simulink model "abssq06alg_fixpt8_32"  (R2021b)
settings: Solver=VariableStepAuto  StartTime=0.0  StopTime=99  RelTol=1e-3
undefined symbols (not defined in the file or in its folder): S, vsva2197, xcvc1902
libraries: hdlBasic x800, vmcUtilities x1
(part 1 of 6)
settings Model: Creator=abeshu  LastModifiedBy=shu_abe

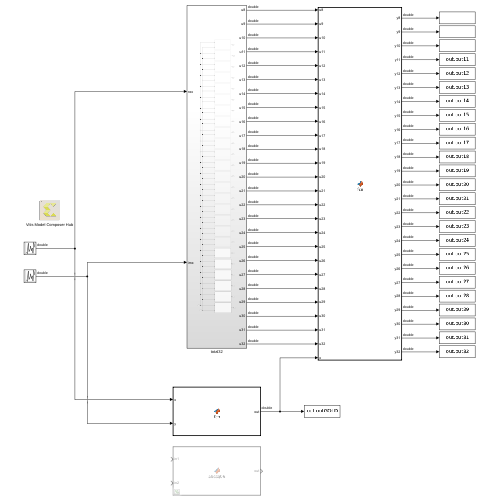
[thumbnail: Simulink's stored preview of the top-level diagram]
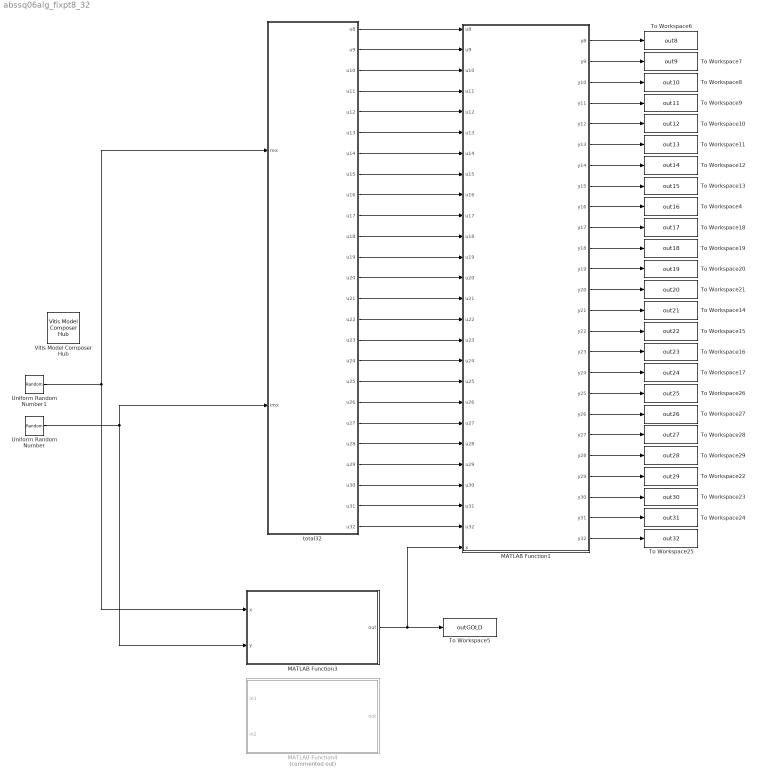
== system abssq06alg_fixpt8_32 ==
  MATLAB Function1 : MATLAB Function  TreatAsAtomicUnit=on
  MATLAB Function3 : MATLAB Function  TreatAsAtomicUnit=on
  MATLAB Function4 : MATLAB Function  Commented=on  TreatAsAtomicUnit=on
  To Workspace10 : ToWorkspace  VariableName=out12  SaveFormat=Structure With Time  SampleTime=-1
  To Workspace11 : ToWorkspace  VariableName=out13  SaveFormat=Structure With Time  SampleTime=-1
  To Workspace12 : ToWorkspace  VariableName=out14  SaveFormat=Structure With Time  SampleTime=-1
  To Workspace13 : ToWorkspace  VariableName=out15  SaveFormat=Structure With Time  SampleTime=-1
  To Workspace14 : ToWorkspace  VariableName=out21  SaveFormat=Structure With Time  SampleTime=-1
  To Workspace15 : ToWorkspace  VariableName=out22  SaveFormat=Structure With Time  SampleTime=-1
  To Workspace16 : ToWorkspace  VariableName=out23  SaveFormat=Structure With Time  SampleTime=-1
  To Workspace17 : ToWorkspace  VariableName=out24  SaveFormat=Structure With Time  SampleTime=-1
  To Workspace18 : ToWorkspace  VariableName=out17  SaveFormat=Structure With Time  SampleTime=-1
  To Workspace19 : ToWorkspace  VariableName=out18  SaveFormat=Structure With Time  SampleTime=-1
  To Workspace20 : ToWorkspace  VariableName=out19  SaveFormat=Structure With Time  SampleTime=-1
  To Workspace21 : ToWorkspace  VariableName=out20  SaveFormat=Structure With Time  SampleTime=-1
  To Workspace22 : ToWorkspace  VariableName=out29  SaveFormat=Structure With Time  SampleTime=-1
  To Workspace23 : ToWorkspace  VariableName=out30  SaveFormat=Structure With Time  SampleTime=-1
  To Workspace24 : ToWorkspace  VariableName=out31  SaveFormat=Structure With Time  SampleTime=-1
  To Workspace25 : ToWorkspace  VariableName=out32  SaveFormat=Structure With Time  SampleTime=-1
  To Workspace26 : ToWorkspace  VariableName=out25  SaveFormat=Structure With Time  SampleTime=-1
  To Workspace27 : ToWorkspace  VariableName=out26  SaveFormat=Structure With Time  SampleTime=-1
  To Workspace28 : ToWorkspace  VariableName=out27  SaveFormat=Structure With Time  SampleTime=-1
  To Workspace29 : ToWorkspace  VariableName=out28  SaveFormat=Structure With Time  SampleTime=-1
  To Workspace4 : ToWorkspace  VariableName=out16  SaveFormat=Structure With Time  SampleTime=-1
  To Workspace5 : ToWorkspace  VariableName=outGOLD  SaveFormat=Structure With Time  SampleTime=-1
  To Workspace6 : ToWorkspace  VariableName=out8  SaveFormat=Structure With Time  SampleTime=-1
  To Workspace7 : ToWorkspace  VariableName=out9  SaveFormat=Structure With Time  SampleTime=-1
  To Workspace8 : ToWorkspace  VariableName=out10  SaveFormat=Structure With Time  SampleTime=-1
  To Workspace9 : ToWorkspace  VariableName=out11  SaveFormat=Structure With Time  SampleTime=-1
  Uniform Random Number : UniformRandomNumber  Minimum=-0.9  Maximum=0.9  SampleTime=1
  Uniform Random Number1 : UniformRandomNumber  Minimum=-0.9  Maximum=0.9  Seed=1  SampleTime=1
  Vitis Model Composer Hub : vmcUtilities/Vitis Model Composer Hub  Tag=genX  CodeGeneration=off  SubsystemName=<enter or select subsystem name>  TargetDirectory=./code  ExportType=HLS C++ code  IpVendor=xilinx.com  IpLibrary=hls  IpVersion=1.0  IpHWLanguage=Verilog  AieCompilerOptions={}  CreateTestbench=off  TestbenchStackSize=10  RunAieSim=off  AieSimTimeout=50000  RunAieSimProfiling=off  LaunchVitisAnalyzer=off  PlotOutput=off  RunX86Sim=off  X86SimTimeout=10  GenHwImage=off  PlatformType=Not Specified  HwSystemType=Baremetal  HwValidationTarget=hw  ProjDevice=Alveo U250 Data Center Accelerator Card (xcu250-figd2104-2L-e)  ProjDevicePart=xcvc1902-vsva2197-2MP-e-S  SamplePeriod=-1  ClockFrequency=200  DataPathParallelism=1  xilinxfamily=virtexuplus  part=xcu250  speed=-2L-e  package=figd2104  directory=./abssq06alg_fixpt27_32  testbench=off  incr_netlist=off  synthesis_tool=Vivado  clock_wrapper=Clock Enables  dbl_ovrd=According to Block Masks  dcm_input_clock_period=10  sysclk_period=50  simulink_period=1  eval_field=0
  total32 : Subsystem
  wires:
  MATLAB Function3/1(out) -> MATLAB Function1/26(x), To Workspace5/1
  Uniform Random Number1/1 -> MATLAB Function3/1(x), total32/1(rex)
  Uniform Random Number/1 -> MATLAB Function3/2(y), total32/2(imx)
  MATLAB Function1/14(y21) -> To Workspace14/1
  MATLAB Function1/3(y10) -> To Workspace8/1
  MATLAB Function1/1(y8) -> To Workspace6/1
  MATLAB Function1/23(y30) -> To Workspace23/1
  MATLAB Function1/12(y19) -> To Workspace20/1
  MATLAB Function1/21(y28) -> To Workspace29/1
  MATLAB Function1/15(y22) -> To Workspace15/1
  MATLAB Function1/4(y11) -> To Workspace9/1
  MATLAB Function1/7(y14) -> To Workspace12/1
  MATLAB Function1/24(y31) -> To Workspace24/1
  MATLAB Function1/2(y9) -> To Workspace7/1
  MATLAB Function1/8(y15) -> To Workspace13/1
  MATLAB Function1/6(y13) -> To Workspace11/1
  MATLAB Function1/5(y12) -> To Workspace10/1
  MATLAB Function1/11(y18) -> To Workspace19/1
  MATLAB Function1/25(y32) -> To Workspace25/1
  MATLAB Function1/13(y20) -> To Workspace21/1
  MATLAB Function1/22(y29) -> To Workspace22/1
  MATLAB Function1/19(y26) -> To Workspace27/1
  MATLAB Function1/16(y23) -> To Workspace16/1
  MATLAB Function1/9(y16) -> To Workspace4/1
  MATLAB Function1/10(y17) -> To Workspace18/1
  MATLAB Function1/17(y24) -> To Workspace17/1
  MATLAB Function1/18(y25) -> To Workspace26/1
  MATLAB Function1/20(y27) -> To Workspace28/1
  total32/1(u8) -> MATLAB Function1/1(u8)
  total32/2(u9) -> MATLAB Function1/2(u9)
  total32/3(u10) -> MATLAB Function1/3(u10)
  total32/4(u11) -> MATLAB Function1/4(u11)
  total32/5(u12) -> MATLAB Function1/5(u12)
  total32/6(u13) -> MATLAB Function1/6(u13)
  total32/7(u14) -> MATLAB Function1/7(u14)
  total32/8(u15) -> MATLAB Function1/8(u15)
  total32/9(u16) -> MATLAB Function1/9(u16)
  total32/10(u17) -> MATLAB Function1/10(u17)
  total32/11(u18) -> MATLAB Function1/11(u18)
  total32/12(u19) -> MATLAB Function1/12(u19)
  total32/13(u20) -> MATLAB Function1/13(u20)
  total32/14(u21) -> MATLAB Function1/14(u21)
  total32/15(u22) -> MATLAB Function1/15(u22)
  total32/16(u23) -> MATLAB Function1/16(u23)
  total32/17(u24) -> MATLAB Function1/17(u24)
  total32/18(u25) -> MATLAB Function1/18(u25)
  total32/19(u26) -> MATLAB Function1/19(u26)
  total32/20(u27) -> MATLAB Function1/20(u27)
  total32/21(u28) -> MATLAB Function1/21(u28)
  total32/22(u29) -> MATLAB Function1/22(u29)
  total32/23(u30) -> MATLAB Function1/23(u30)
  total32/24(u31) -> MATLAB Function1/24(u31)
  total32/25(u32) -> MATLAB Function1/25(u32)

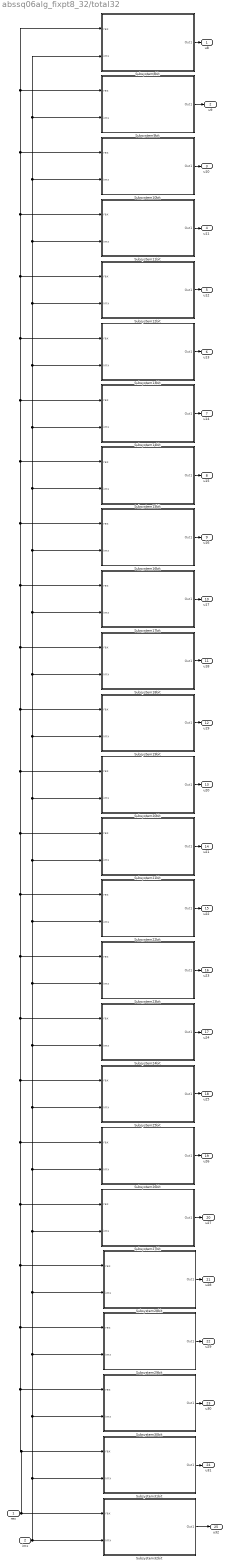
== system abssq06alg_fixpt8_32/total32 ==
  rex : Inport
  imx : Inport  Port=2
  Subsystem10bit : Subsystem
      mask Display: %%%%
  Subsystem11bit : Subsystem
      mask Display: %%%%
  Subsystem12bit : Subsystem
      mask Display: %%%%
  Subsystem13bit : Subsystem
      mask Display: %%%%
  Subsystem14bit : Subsystem
      mask Display: %%%%
  Subsystem15bit : Subsystem
      mask Display: %%%%
  Subsystem16bit : Subsystem
      mask Display: %%%%
  Subsystem17bit : Subsystem
      mask Display: %%%%
  Subsystem18bit : Subsystem
      mask Display: %%%%
  Subsystem19bit : Subsystem
      mask Display: %%%%
  Subsystem20bit : Subsystem
      mask Display: %%%%
  Subsystem21bit : Subsystem
      mask Display: %%%%
  Subsystem22bit : Subsystem
      mask Display: %%%%
  Subsystem23bit : Subsystem
      mask Display: %%%%
  Subsystem24bit : Subsystem
      mask Display: %%%%
  Subsystem25bit : Subsystem
      mask Display: %%%%
  Subsystem26bit : Subsystem
      mask Display: %%%%
  Subsystem27bit : Subsystem
      mask Display: %%%%
  Subsystem28bit : Subsystem
      mask Display: %%%%
  Subsystem29bit : Subsystem
      mask Display: %%%%
  Subsystem30bit : Subsystem
      mask Display: %%%%
  Subsystem31bit : Subsystem
      mask Display: %%%%
  Subsystem32bit : Subsystem
      mask Display: %%%%
  Subsystem8bit : Subsystem
      mask Display: %%%%
  Subsystem9bit : Subsystem
      mask Display: %%%%
  u8 : Outport
  u9 : Outport  Port=2
  u10 : Outport  Port=3
  u11 : Outport  Port=4
  u12 : Outport  Port=5
  u13 : Outport  Port=6
  u14 : Outport  Port=7
  u15 : Outport  Port=8
  u16 : Outport  Port=9
  u17 : Outport  Port=10
  u18 : Outport  Port=11
  u19 : Outport  Port=12
  u20 : Outport  Port=13
  u21 : Outport  Port=14
  u22 : Outport  Port=15
  u23 : Outport  Port=16
  u24 : Outport  Port=17
  u25 : Outport  Port=18
  u26 : Outport  Port=19
  u27 : Outport  Port=20
  u28 : Outport  Port=21
  u29 : Outport  Port=22
  u30 : Outport  Port=23
  u31 : Outport  Port=24
  u32 : Outport  Port=25
  wires:
  Subsystem17bit/1(Out1) -> u17/1
  Subsystem30bit/1(Out1) -> u30/1
  Subsystem15bit/1(Out1) -> u15/1
  Subsystem12bit/1(Out1) -> u12/1
  Subsystem14bit/1(Out1) -> u14/1
  Subsystem28bit/1(Out1) -> u28/1
  Subsystem22bit/1(Out1) -> u22/1
  Subsystem13bit/1(Out1) -> u13/1
  Subsystem21bit/1(Out1) -> u21/1
  rex/1 -> Subsystem32bit/1(rex), Subsystem31bit/1(rex), Subsystem30bit/1(rex), Subsystem29bit/1(rex), Subsystem28bit/1(rex), Subsystem27bit/1(rex), Subsystem26bit/1(rex), Subsystem25bit/1(rex), Subsystem24bit/1(rex), Subsystem23bit/1(rex), Subsystem22bit/1(rex), Subsystem21bit/1(rex), Subsystem20bit/1(rex), Subsystem19bit/1(rex), Subsystem18bit/1(rex), Subsystem17bit/1(rex), Subsystem16bit/1(rex), Subsystem15bit/1(rex), Subsystem14bit/1(rex), Subsystem13bit/1(rex), Subsystem12bit/1(rex), Subsystem11bit/1(rex), Subsystem10bit/1(rex), Subsystem9bit/1(rex), Subsystem8bit/1(rex)
  Subsystem26bit/1(Out1) -> u26/1
  Subsystem19bit/1(Out1) -> u19/1
  Subsystem10bit/1(Out1) -> u10/1
  Subsystem11bit/1(Out1) -> u11/1
  Subsystem25bit/1(Out1) -> u25/1
  Subsystem18bit/1(Out1) -> u18/1
  Subsystem20bit/1(Out1) -> u20/1
  Subsystem23bit/1(Out1) -> u23/1
  Subsystem16bit/1(Out1) -> u16/1
  Subsystem32bit/1(Out1) -> u32/1
  Subsystem27bit/1(Out1) -> u27/1
  Subsystem31bit/1(Out1) -> u31/1
  Subsystem29bit/1(Out1) -> u29/1
  Subsystem24bit/1(Out1) -> u24/1
  Subsystem8bit/1(Out1) -> u8/1
  imx/1 -> Subsystem32bit/2(imx), Subsystem31bit/2(imx), Subsystem30bit/2(imx), Subsystem29bit/2(imx), Subsystem28bit/2(imx), Subsystem27bit/2(imx), Subsystem26bit/2(imx), Subsystem25bit/2(imx), Subsystem24bit/2(imx), Subsystem23bit/2(imx), Subsystem22bit/2(imx), Subsystem21bit/2(imx), Subsystem20bit/2(imx), Subsystem19bit/2(imx), Subsystem18bit/2(imx), Subsystem17bit/2(imx), Subsystem16bit/2(imx), Subsystem15bit/2(imx), Subsystem14bit/2(imx), Subsystem13bit/2(imx), Subsystem12bit/2(imx), Subsystem11bit/2(imx), Subsystem10bit/2(imx), Subsystem9bit/2(imx), Subsystem8bit/2(imx)
  Subsystem9bit/1(Out1) -> u9/1

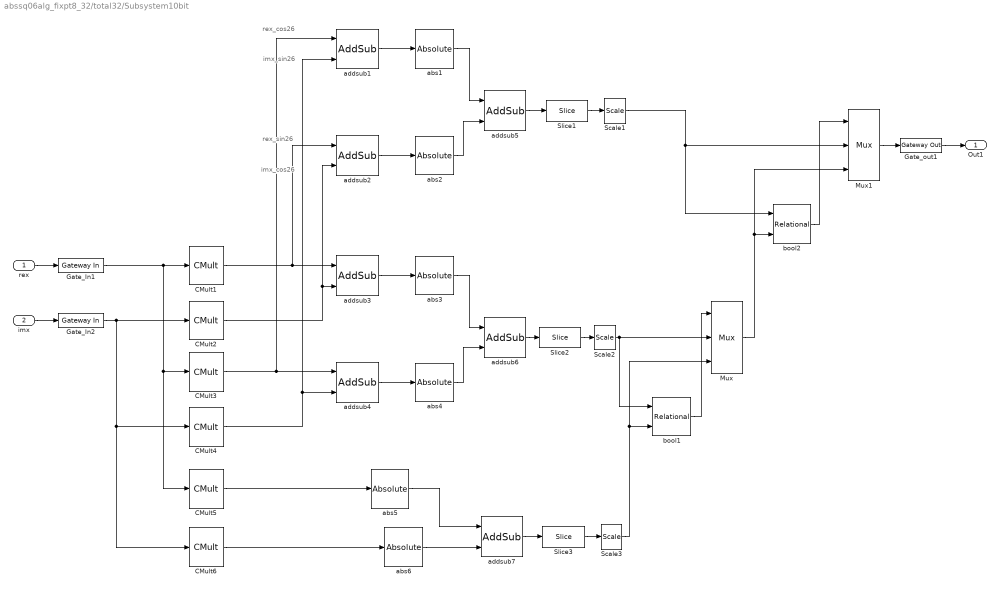
== system abssq06alg_fixpt8_32/total32/Subsystem10bit ==
  note: imx_cos26
  note: rex_sin26
  note: imx_sin26
  note: rex_cos26
  rex : Inport
  imx : Inport  Port=2
  CMult1 : hdlBasic/CMult  const=1/sqrt(2)*cos(pi/6)  gui_display_data_type=Fixed-point  const_n_bits=10  const_bin_pt=9  float_type=Double  exp_bits=8  fraction_bits=24  en=off  latency=0  precision=Full  arith_type="Signed  (2's comp)"  n_bits=16  bin_pt=14  quantization=Truncate  overflow=Wrap  use_behavioral_HDL=off  mem_type=Distributed RAM  pipeline=off  XmcBlockStatus=1  maskContainerNames=tabcontainer1  block_type=cmult  block_config=sysgen:CMult_config
      settings: infoedit=[]
  CMult2 : hdlBasic/CMult  const=1/sqrt(2)*sin(pi/6)  gui_display_data_type=Fixed-point  const_n_bits=10  const_bin_pt=9  float_type=Double  exp_bits=8  fraction_bits=24  en=off  latency=0  precision=Full  arith_type="Signed  (2's comp)"  n_bits=16  bin_pt=14  quantization=Truncate  overflow=Wrap  use_behavioral_HDL=off  mem_type=Distributed RAM  pipeline=off  XmcBlockStatus=1  maskContainerNames=tabcontainer1  block_type=cmult  block_config=sysgen:CMult_config
      settings: infoedit=[]
  CMult3 : hdlBasic/CMult  const=1/sqrt(2)*sin(pi/6)  gui_display_data_type=Fixed-point  const_n_bits=10  const_bin_pt=9  float_type=Double  exp_bits=8  fraction_bits=24  en=off  latency=0  precision=Full  arith_type="Signed  (2's comp)"  n_bits=16  bin_pt=14  quantization=Truncate  overflow=Wrap  use_behavioral_HDL=off  mem_type=Distributed RAM  pipeline=off  XmcBlockStatus=1  maskContainerNames=tabcontainer1  block_type=cmult  block_config=sysgen:CMult_config
      settings: infoedit=[]
  CMult4 : hdlBasic/CMult  const=1/sqrt(2)*cos(pi/6)  gui_display_data_type=Fixed-point  const_n_bits=10  const_bin_pt=9  float_type=Double  exp_bits=8  fraction_bits=24  en=off  latency=0  precision=Full  arith_type="Signed  (2's comp)"  n_bits=16  bin_pt=14  quantization=Truncate  overflow=Wrap  use_behavioral_HDL=off  mem_type=Distributed RAM  pipeline=off  XmcBlockStatus=1  maskContainerNames=tabcontainer1  block_type=cmult  block_config=sysgen:CMult_config
      settings: infoedit=[]
  CMult5 : hdlBasic/CMult  const=1/sqrt(2)  gui_display_data_type=Fixed-point  const_n_bits=10  const_bin_pt=9  float_type=Double  exp_bits=8  fraction_bits=24  en=off  latency=0  precision=Full  arith_type="Signed  (2's comp)"  n_bits=16  bin_pt=14  quantization=Truncate  overflow=Wrap  use_behavioral_HDL=off  mem_type=Distributed RAM  pipeline=off  XmcBlockStatus=1  maskContainerNames=tabcontainer1  block_type=cmult  block_config=sysgen:CMult_config
      settings: infoedit=[]
  CMult6 : hdlBasic/CMult  const=1/sqrt(2)  gui_display_data_type=Fixed-point  const_n_bits=10  const_bin_pt=9  float_type=Double  exp_bits=8  fraction_bits=24  en=off  latency=0  precision=Full  arith_type="Signed  (2's comp)"  n_bits=16  bin_pt=14  quantization=Truncate  overflow=Wrap  use_behavioral_HDL=off  mem_type=Distributed RAM  pipeline=off  XmcBlockStatus=1  maskContainerNames=tabcontainer1  block_type=cmult  block_config=sysgen:CMult_config
      settings: infoedit=[]
  Gate_In1 : hdlBasic/Gateway In  gui_display_data_type=Fixed-point  arith_type=Signed (2's comp)  n_bits=10  bin_pt=8  preci_type=Double  exp_width=8  frac_width=24  rows=1  columns=1  quantization="Round  (unbiased: +/- Inf)"  overflow=Saturate  period=1  UseAsADC=off  ADCChannel='1'  interface=None  automatic_assignment=on  address_offset=hex2dec('00')  intf_name=''  intf_description=''  default_value=0  timing_constraint=None  locs_specified=off  LOCs={}  io_standard={}  inherit_from_input=off  hdl_port=on  XmcBlockStatus=1  maskContainerNames=group4  block_type=gatewayin  block_config=sysgen:gateway_in_config  block_width_w=590  block_height_w=620  block_width=640  block_height=850
  Gate_In2 : hdlBasic/Gateway In  gui_display_data_type=Fixed-point  arith_type=Signed (2's comp)  n_bits=10  bin_pt=8  preci_type=Double  exp_width=8  frac_width=24  rows=1  columns=1  quantization="Round  (unbiased: +/- Inf)"  overflow=Saturate  period=1  UseAsADC=off  ADCChannel='1'  interface=None  automatic_assignment=on  address_offset=hex2dec('00')  intf_name=''  intf_description=''  default_value=0  timing_constraint=None  locs_specified=off  LOCs={}  io_standard={}  inherit_from_input=off  hdl_port=on  XmcBlockStatus=1  maskContainerNames=group4  block_type=gatewayin  block_config=sysgen:gateway_in_config  block_width_w=590  block_height_w=620  block_width=640  block_height=850
  Gate_out1 : hdlBasic/Gateway Out  inherit_from_input=off  hdl_port=on  rows=1  columns=1  UseAsDAC=off  DACChannel='1'  interface=None  automatic_assignment=on  address_offset=hex2dec('00')  intf_name=''  intf_description=''  timing_constraint=None  locs_specified=off  LOCs={}  io_standard={}  XmcBlockStatus=1  maskContainerNames=group4  block_type=gatewayout  block_config=sysgen:gateway_out_config  block_width_w=590  block_height_w=620  block_width=620  block_height=750
  Mux : hdlBasic/Mux  inputs=2  en=off  latency=0  precision=Full  arith_type=Unsigned  n_bits=16  bin_pt=14  quantization=Truncate  overflow=Wrap  XmcBlockStatus=1  maskContainerNames=tabcontainer1  block_type=mux  block_config=sysgen:Mux_config
  Mux1 : hdlBasic/Mux  inputs=2  en=off  latency=0  precision=Full  arith_type=Unsigned  n_bits=16  bin_pt=14  quantization=Truncate  overflow=Wrap  XmcBlockStatus=1  maskContainerNames=tabcontainer1  block_type=mux  block_config=sysgen:Mux_config
  Scale1 : hdlBasic/Scale  scale_factor=-9  XmcBlockStatus=1  maskContainerNames=group1  block_type=scale  block_config=sysgen:Scale_config
  Scale2 : hdlBasic/Scale  scale_factor=-9  XmcBlockStatus=1  maskContainerNames=group1  block_type=scale  block_config=sysgen:Scale_config
  Scale3 : hdlBasic/Scale  scale_factor=-9  XmcBlockStatus=1  maskContainerNames=group1  block_type=scale  block_config=sysgen:Scale_config
  Slice1 : hdlBasic/Slice  nbits=7  boolean_output=off  mode=Two Bit Locations  bit1=-5  base1=MSB of Input  bit0=8  base0=LSB of Input  XmcBlockStatus=1  maskContainerNames=group1  block_type=slice  block_config=sysgen:Slice_config
  Slice2 : hdlBasic/Slice  nbits=7  boolean_output=off  mode=Two Bit Locations  bit1=-5  base1=MSB of Input  bit0=8  base0=LSB of Input  XmcBlockStatus=1  maskContainerNames=group1  block_type=slice  block_config=sysgen:Slice_config
  Slice3 : hdlBasic/Slice  nbits=10  boolean_output=off  mode=Upper Bit Location + Width  bit1=-4  base1=MSB of Input  bit0=7  base0=LSB of Input  XmcBlockStatus=1  maskContainerNames=group1  block_type=slice  block_config=sysgen:Slice_config
  abs{1..6} (6 alike) : hdlBasic/Absolute  precision=Full  arith_type=Unsigned  n_bits=16  bin_pt=14  quantization=Truncate  overflow=Wrap  en=off  latency=0  XmcBlockStatus=1  maskContainerNames=tabcontainer1  block_type=abs  block_config=sysgen:Abs_config
  addsub1 : hdlBasic/AddSub  mode=Subtraction  use_carryin=off  use_carryout=off  en=off  latency=0  precision=Full  arith_type="Signed  (2's comp)"  n_bits=35  bin_pt=32  quantization="Round  (unbiased: +/- Inf)"  overflow=Saturate  use_behavioral_HDL=off  hw_selection=Fabric  pipelined=on  XmcBlockStatus=1  maskContainerNames=tabcontainer1  block_type=addsub  block_config=sysgen:Addsub_config
  addsub{2,4..6} (4 alike) : hdlBasic/AddSub  mode=Addition  use_carryin=off  use_carryout=off  en=off  latency=0  precision=Full  arith_type=Unsigned  n_bits=16  bin_pt=14  quantization="Round  (unbiased: +/- Inf)"  overflow=Saturate  use_behavioral_HDL=off  hw_selection=Fabric  pipelined=on  XmcBlockStatus=1  maskContainerNames=tabcontainer1  block_type=addsub  block_config=sysgen:Addsub_config
  addsub3 : hdlBasic/AddSub  mode=Subtraction  use_carryin=off  use_carryout=off  en=off  latency=0  precision=Full  arith_type="Signed  (2's comp)"  n_bits=35  bin_pt=32  quantization="Round  (unbiased: +/- Inf)"  overflow=Saturate  use_behavioral_HDL=off  hw_selection=Fabric  pipelined=on  XmcBlockStatus=1  maskContainerNames=tabcontainer1  block_type=addsub  block_config=sysgen:Addsub_config
  addsub7 : hdlBasic/AddSub  mode=Addition  use_carryin=off  use_carryout=off  en=off  latency=0  precision=Full  arith_type=Unsigned  n_bits=17  bin_pt=16  quantization="Round  (unbiased: +/- Inf)"  overflow=Saturate  use_behavioral_HDL=off  hw_selection=Fabric  pipelined=on  XmcBlockStatus=1  maskContainerNames=tabcontainer1  block_type=addsub  block_config=sysgen:Addsub_config
  bool1 : hdlBasic/Relational  mode=a<b  op_type=Bool  en=off  latency=0  XmcBlockStatus=1  maskContainerNames=tabcontainer1  block_type=relational  block_config=sysgen:Relational_config
  bool2 : hdlBasic/Relational  mode=a<b  op_type=Bool  en=off  latency=0  XmcBlockStatus=1  maskContainerNames=tabcontainer1  block_type=relational  block_config=sysgen:Relational_config
  Out1 : Outport
  wires:
  addsub3/1 -> abs3/1
  abs3/1 -> addsub6/1
  CMult1/1 -> addsub3/1, addsub2/1
  CMult2/1 -> addsub2/2, addsub3/2
  imx/1 -> Gate_In2/1
  rex/1 -> Gate_In1/1
  bool1/1 -> Mux/1
  addsub4/1 -> abs4/1
  abs4/1 -> addsub6/2
  Gate_In1/1 -> CMult1/1, CMult5/1, CMult3/1
  Gate_In2/1 -> CMult4/1, CMult6/1, CMult2/1
  CMult3/1 -> addsub4/1, addsub1/1
  CMult4/1 -> addsub4/2, addsub1/2
  addsub2/1 -> abs2/1
  abs2/1 -> addsub5/2
  addsub1/1 -> abs1/1
  abs1/1 -> addsub5/1
  Gate_out1/1 -> Out1/1
  Scale1/1 -> bool2/1, Mux1/2
  Mux/1 -> Mux1/3, bool2/2
  bool2/1 -> Mux1/1
  abs5/1 -> addsub7/1
  abs6/1 -> addsub7/2
  Mux1/1 -> Gate_out1/1
  Slice2/1 -> Scale2/1
  Slice1/1 -> Scale1/1
  Slice3/1 -> Scale3/1
  Scale2/1 -> bool1/1, Mux/2
  Scale3/1 -> Mux/3, bool1/2
  CMult5/1 -> abs5/1
  CMult6/1 -> abs6/1
  addsub5/1 -> Slice1/1
  addsub6/1 -> Slice2/1
  addsub7/1 -> Slice3/1

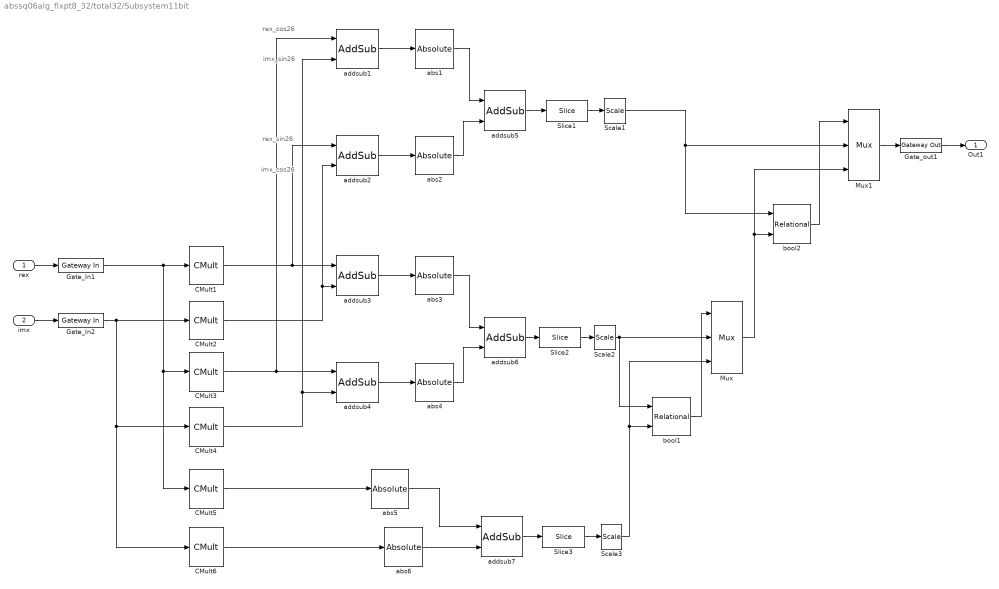
== system abssq06alg_fixpt8_32/total32/Subsystem11bit ==
  note: imx_cos26
  note: rex_sin26
  note: imx_sin26
  note: rex_cos26
  rex : Inport
  imx : Inport  Port=2
  CMult1 : hdlBasic/CMult  const=1/sqrt(2)*cos(pi/6)  gui_display_data_type=Fixed-point  const_n_bits=11  const_bin_pt=10  float_type=Double  exp_bits=8  fraction_bits=24  en=off  latency=0  precision=Full  arith_type="Signed  (2's comp)"  n_bits=16  bin_pt=14  quantization=Truncate  overflow=Wrap  use_behavioral_HDL=off  mem_type=Distributed RAM  pipeline=off  XmcBlockStatus=1  maskContainerNames=tabcontainer1  block_type=cmult  block_config=sysgen:CMult_config
      settings: infoedit=[]
  CMult2 : hdlBasic/CMult  const=1/sqrt(2)*sin(pi/6)  gui_display_data_type=Fixed-point  const_n_bits=11  const_bin_pt=10  float_type=Double  exp_bits=8  fraction_bits=24  en=off  latency=0  precision=Full  arith_type="Signed  (2's comp)"  n_bits=16  bin_pt=14  quantization=Truncate  overflow=Wrap  use_behavioral_HDL=off  mem_type=Distributed RAM  pipeline=off  XmcBlockStatus=1  maskContainerNames=tabcontainer1  block_type=cmult  block_config=sysgen:CMult_config
      settings: infoedit=[]
  CMult3 : hdlBasic/CMult  const=1/sqrt(2)*sin(pi/6)  gui_display_data_type=Fixed-point  const_n_bits=11  const_bin_pt=10  float_type=Double  exp_bits=8  fraction_bits=24  en=off  latency=0  precision=Full  arith_type="Signed  (2's comp)"  n_bits=16  bin_pt=14  quantization=Truncate  overflow=Wrap  use_behavioral_HDL=off  mem_type=Distributed RAM  pipeline=off  XmcBlockStatus=1  maskContainerNames=tabcontainer1  block_type=cmult  block_config=sysgen:CMult_config
      settings: infoedit=[]
  CMult4 : hdlBasic/CMult  const=1/sqrt(2)*cos(pi/6)  gui_display_data_type=Fixed-point  const_n_bits=11  const_bin_pt=10  float_type=Double  exp_bits=8  fraction_bits=24  en=off  latency=0  precision=Full  arith_type="Signed  (2's comp)"  n_bits=16  bin_pt=14  quantization=Truncate  overflow=Wrap  use_behavioral_HDL=off  mem_type=Distributed RAM  pipeline=off  XmcBlockStatus=1  maskContainerNames=tabcontainer1  block_type=cmult  block_config=sysgen:CMult_config
      settings: infoedit=[]
  CMult5 : hdlBasic/CMult  const=1/sqrt(2)  gui_display_data_type=Fixed-point  const_n_bits=11  const_bin_pt=10  float_type=Double  exp_bits=8  fraction_bits=24  en=off  latency=0  precision=Full  arith_type="Signed  (2's comp)"  n_bits=16  bin_pt=14  quantization=Truncate  overflow=Wrap  use_behavioral_HDL=off  mem_type=Distributed RAM  pipeline=off  XmcBlockStatus=1  maskContainerNames=tabcontainer1  block_type=cmult  block_config=sysgen:CMult_config
      settings: infoedit=[]
  CMult6 : hdlBasic/CMult  const=1/sqrt(2)  gui_display_data_type=Fixed-point  const_n_bits=11  const_bin_pt=10  float_type=Double  exp_bits=8  fraction_bits=24  en=off  latency=0  precision=Full  arith_type="Signed  (2's comp)"  n_bits=16  bin_pt=14  quantization=Truncate  overflow=Wrap  use_behavioral_HDL=off  mem_type=Distributed RAM  pipeline=off  XmcBlockStatus=1  maskContainerNames=tabcontainer1  block_type=cmult  block_config=sysgen:CMult_config
      settings: infoedit=[]
  Gate_In1 : hdlBasic/Gateway In  gui_display_data_type=Fixed-point  arith_type=Signed (2's comp)  n_bits=11  bin_pt=9  preci_type=Double  exp_width=8  frac_width=24  rows=1  columns=1  quantization="Round  (unbiased: +/- Inf)"  overflow=Saturate  period=1  UseAsADC=off  ADCChannel='1'  interface=None  automatic_assignment=on  address_offset=hex2dec('00')  intf_name=''  intf_description=''  default_value=0  timing_constraint=None  locs_specified=off  LOCs={}  io_standard={}  inherit_from_input=off  hdl_port=on  XmcBlockStatus=1  maskContainerNames=group4  block_type=gatewayin  block_config=sysgen:gateway_in_config  block_width_w=590  block_height_w=620  block_width=640  block_height=850
  Gate_In2 : hdlBasic/Gateway In  gui_display_data_type=Fixed-point  arith_type=Signed (2's comp)  n_bits=11  bin_pt=9  preci_type=Double  exp_width=8  frac_width=24  rows=1  columns=1  quantization="Round  (unbiased: +/- Inf)"  overflow=Saturate  period=1  UseAsADC=off  ADCChannel='1'  interface=None  automatic_assignment=on  address_offset=hex2dec('00')  intf_name=''  intf_description=''  default_value=0  timing_constraint=None  locs_specified=off  LOCs={}  io_standard={}  inherit_from_input=off  hdl_port=on  XmcBlockStatus=1  maskContainerNames=group4  block_type=gatewayin  block_config=sysgen:gateway_in_config  block_width_w=590  block_height_w=620  block_width=640  block_height=850
  Gate_out1 : hdlBasic/Gateway Out  inherit_from_input=off  hdl_port=on  rows=1  columns=1  UseAsDAC=off  DACChannel='1'  interface=None  automatic_assignment=on  address_offset=hex2dec('00')  intf_name=''  intf_description=''  timing_constraint=None  locs_specified=off  LOCs={}  io_standard={}  XmcBlockStatus=1  maskContainerNames=group4  block_type=gatewayout  block_config=sysgen:gateway_out_config  block_width_w=590  block_height_w=620  block_width=620  block_height=750
  Mux : hdlBasic/Mux  inputs=2  en=off  latency=0  precision=Full  arith_type=Unsigned  n_bits=16  bin_pt=14  quantization=Truncate  overflow=Wrap  XmcBlockStatus=1  maskContainerNames=tabcontainer1  block_type=mux  block_config=sysgen:Mux_config
  Mux1 : hdlBasic/Mux  inputs=2  en=off  latency=0  precision=Full  arith_type=Unsigned  n_bits=16  bin_pt=14  quantization=Truncate  overflow=Wrap  XmcBlockStatus=1  maskContainerNames=tabcontainer1  block_type=mux  block_config=sysgen:Mux_config
  Scale1 : hdlBasic/Scale  scale_factor=-10  XmcBlockStatus=1  maskContainerNames=group1  block_type=scale  block_config=sysgen:Scale_config
  Scale2 : hdlBasic/Scale  scale_factor=-10  XmcBlockStatus=1  maskContainerNames=group1  block_type=scale  block_config=sysgen:Scale_config
  Scale3 : hdlBasic/Scale  scale_factor=-10  XmcBlockStatus=1  maskContainerNames=group1  block_type=scale  block_config=sysgen:Scale_config
  Slice1 : hdlBasic/Slice  nbits=7  boolean_output=off  mode=Two Bit Locations  bit1=-5  base1=MSB of Input  bit0=9  base0=LSB of Input  XmcBlockStatus=1  maskContainerNames=group1  block_type=slice  block_config=sysgen:Slice_config
  Slice2 : hdlBasic/Slice  nbits=7  boolean_output=off  mode=Two Bit Locations  bit1=-5  base1=MSB of Input  bit0=9  base0=LSB of Input  XmcBlockStatus=1  maskContainerNames=group1  block_type=slice  block_config=sysgen:Slice_config
  Slice3 : hdlBasic/Slice  nbits=11  boolean_output=off  mode=Upper Bit Location + Width  bit1=-4  base1=MSB of Input  bit0=7  base0=LSB of Input  XmcBlockStatus=1  maskContainerNames=group1  block_type=slice  block_config=sysgen:Slice_config
  abs{1..6} (6 alike) : hdlBasic/Absolute  precision=Full  arith_type=Unsigned  n_bits=16  bin_pt=14  quantization=Truncate  overflow=Wrap  en=off  latency=0  XmcBlockStatus=1  maskContainerNames=tabcontainer1  block_type=abs  block_config=sysgen:Abs_config
  addsub1 : hdlBasic/AddSub  mode=Subtraction  use_carryin=off  use_carryout=off  en=off  latency=0  precision=Full  arith_type="Signed  (2's comp)"  n_bits=35  bin_pt=32  quantization="Round  (unbiased: +/- Inf)"  overflow=Saturate  use_behavioral_HDL=off  hw_selection=Fabric  pipelined=on  XmcBlockStatus=1  maskContainerNames=tabcontainer1  block_type=addsub  block_config=sysgen:Addsub_config
  addsub{2,4..6} (4 alike) : hdlBasic/AddSub  mode=Addition  use_carryin=off  use_carryout=off  en=off  latency=0  precision=Full  arith_type=Unsigned  n_bits=16  bin_pt=14  quantization="Round  (unbiased: +/- Inf)"  overflow=Saturate  use_behavioral_HDL=off  hw_selection=Fabric  pipelined=on  XmcBlockStatus=1  maskContainerNames=tabcontainer1  block_type=addsub  block_config=sysgen:Addsub_config
  addsub3 : hdlBasic/AddSub  mode=Subtraction  use_carryin=off  use_carryout=off  en=off  latency=0  precision=Full  arith_type="Signed  (2's comp)"  n_bits=35  bin_pt=32  quantization="Round  (unbiased: +/- Inf)"  overflow=Saturate  use_behavioral_HDL=off  hw_selection=Fabric  pipelined=on  XmcBlockStatus=1  maskContainerNames=tabcontainer1  block_type=addsub  block_config=sysgen:Addsub_config
  addsub7 : hdlBasic/AddSub  mode=Addition  use_carryin=off  use_carryout=off  en=off  latency=0  precision=Full  arith_type=Unsigned  n_bits=17  bin_pt=16  quantization="Round  (unbiased: +/- Inf)"  overflow=Saturate  use_behavioral_HDL=off  hw_selection=Fabric  pipelined=on  XmcBlockStatus=1  maskContainerNames=tabcontainer1  block_type=addsub  block_config=sysgen:Addsub_config
  bool1 : hdlBasic/Relational  mode=a<b  op_type=Bool  en=off  latency=0  XmcBlockStatus=1  maskContainerNames=tabcontainer1  block_type=relational  block_config=sysgen:Relational_config
  bool2 : hdlBasic/Relational  mode=a<b  op_type=Bool  en=off  latency=0  XmcBlockStatus=1  maskContainerNames=tabcontainer1  block_type=relational  block_config=sysgen:Relational_config
  Out1 : Outport
  wires:
  addsub3/1 -> abs3/1
  abs3/1 -> addsub6/1
  CMult1/1 -> addsub3/1, addsub2/1
  CMult2/1 -> addsub2/2, addsub3/2
  imx/1 -> Gate_In2/1
  rex/1 -> Gate_In1/1
  bool1/1 -> Mux/1
  addsub4/1 -> abs4/1
  abs4/1 -> addsub6/2
  Gate_In1/1 -> CMult1/1, CMult5/1, CMult3/1
  Gate_In2/1 -> CMult4/1, CMult6/1, CMult2/1
  CMult3/1 -> addsub4/1, addsub1/1
  CMult4/1 -> addsub4/2, addsub1/2
  addsub2/1 -> abs2/1
  abs2/1 -> addsub5/2
  addsub1/1 -> abs1/1
  abs1/1 -> addsub5/1
  Gate_out1/1 -> Out1/1
  Scale1/1 -> bool2/1, Mux1/2
  Mux/1 -> Mux1/3, bool2/2
  bool2/1 -> Mux1/1
  abs5/1 -> addsub7/1
  abs6/1 -> addsub7/2
  Mux1/1 -> Gate_out1/1
  Slice2/1 -> Scale2/1
  Slice1/1 -> Scale1/1
  Slice3/1 -> Scale3/1
  Scale2/1 -> bool1/1, Mux/2
  Scale3/1 -> Mux/3, bool1/2
  CMult5/1 -> abs5/1
  CMult6/1 -> abs6/1
  addsub5/1 -> Slice1/1
  addsub6/1 -> Slice2/1
  addsub7/1 -> Slice3/1

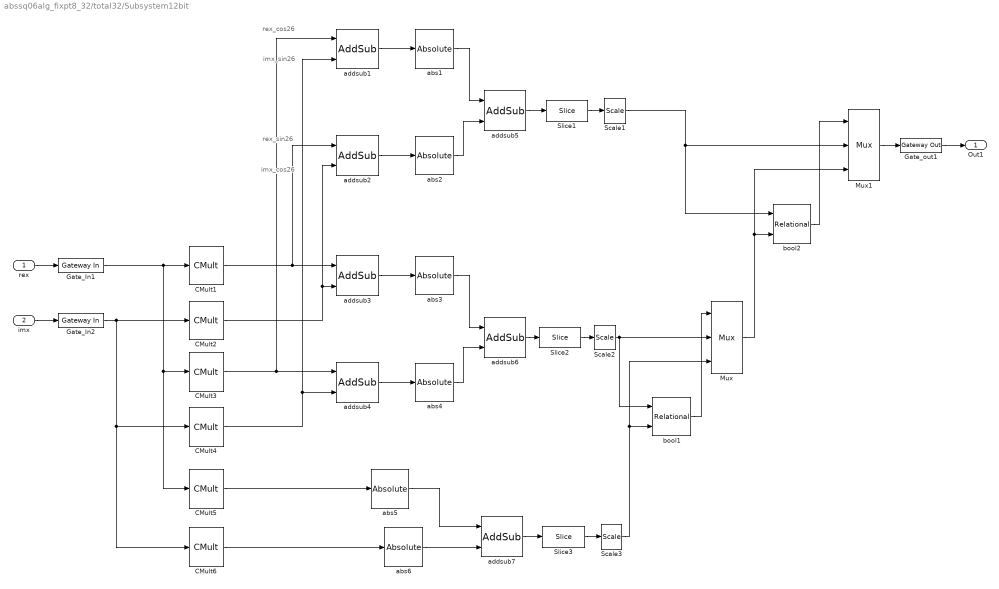
== system abssq06alg_fixpt8_32/total32/Subsystem12bit ==
  note: imx_cos26
  note: rex_sin26
  note: imx_sin26
  note: rex_cos26
  rex : Inport
  imx : Inport  Port=2
  CMult1 : hdlBasic/CMult  const=1/sqrt(2)*cos(pi/6)  gui_display_data_type=Fixed-point  const_n_bits=12  const_bin_pt=11  float_type=Double  exp_bits=8  fraction_bits=24  en=off  latency=0  precision=Full  arith_type="Signed  (2's comp)"  n_bits=16  bin_pt=14  quantization=Truncate  overflow=Wrap  use_behavioral_HDL=off  mem_type=Distributed RAM  pipeline=off  XmcBlockStatus=1  maskContainerNames=tabcontainer1  block_type=cmult  block_config=sysgen:CMult_config
      settings: infoedit=[]
  CMult2 : hdlBasic/CMult  const=1/sqrt(2)*sin(pi/6)  gui_display_data_type=Fixed-point  const_n_bits=12  const_bin_pt=11  float_type=Double  exp_bits=8  fraction_bits=24  en=off  latency=0  precision=Full  arith_type="Signed  (2's comp)"  n_bits=16  bin_pt=14  quantization=Truncate  overflow=Wrap  use_behavioral_HDL=off  mem_type=Distributed RAM  pipeline=off  XmcBlockStatus=1  maskContainerNames=tabcontainer1  block_type=cmult  block_config=sysgen:CMult_config
      settings: infoedit=[]
  CMult3 : hdlBasic/CMult  const=1/sqrt(2)*sin(pi/6)  gui_display_data_type=Fixed-point  const_n_bits=12  const_bin_pt=11  float_type=Double  exp_bits=8  fraction_bits=24  en=off  latency=0  precision=Full  arith_type="Signed  (2's comp)"  n_bits=16  bin_pt=14  quantization=Truncate  overflow=Wrap  use_behavioral_HDL=off  mem_type=Distributed RAM  pipeline=off  XmcBlockStatus=1  maskContainerNames=tabcontainer1  block_type=cmult  block_config=sysgen:CMult_config
      settings: infoedit=[]
  CMult4 : hdlBasic/CMult  const=1/sqrt(2)*cos(pi/6)  gui_display_data_type=Fixed-point  const_n_bits=12  const_bin_pt=11  float_type=Double  exp_bits=8  fraction_bits=24  en=off  latency=0  precision=Full  arith_type="Signed  (2's comp)"  n_bits=16  bin_pt=14  quantization=Truncate  overflow=Wrap  use_behavioral_HDL=off  mem_type=Distributed RAM  pipeline=off  XmcBlockStatus=1  maskContainerNames=tabcontainer1  block_type=cmult  block_config=sysgen:CMult_config
      settings: infoedit=[]
  CMult5 : hdlBasic/CMult  const=1/sqrt(2)  gui_display_data_type=Fixed-point  const_n_bits=12  const_bin_pt=11  float_type=Double  exp_bits=8  fraction_bits=24  en=off  latency=0  precision=Full  arith_type="Signed  (2's comp)"  n_bits=16  bin_pt=14  quantization=Truncate  overflow=Wrap  use_behavioral_HDL=off  mem_type=Distributed RAM  pipeline=off  XmcBlockStatus=1  maskContainerNames=tabcontainer1  block_type=cmult  block_config=sysgen:CMult_config
      settings: infoedit=[]
  CMult6 : hdlBasic/CMult  const=1/sqrt(2)  gui_display_data_type=Fixed-point  const_n_bits=12  const_bin_pt=11  float_type=Double  exp_bits=8  fraction_bits=24  en=off  latency=0  precision=Full  arith_type="Signed  (2's comp)"  n_bits=16  bin_pt=14  quantization=Truncate  overflow=Wrap  use_behavioral_HDL=off  mem_type=Distributed RAM  pipeline=off  XmcBlockStatus=1  maskContainerNames=tabcontainer1  block_type=cmult  block_config=sysgen:CMult_config
      settings: infoedit=[]
  Gate_In1 : hdlBasic/Gateway In  gui_display_data_type=Fixed-point  arith_type=Signed (2's comp)  n_bits=12  bin_pt=10  preci_type=Double  exp_width=8  frac_width=24  rows=1  columns=1  quantization="Round  (unbiased: +/- Inf)"  overflow=Saturate  period=1  UseAsADC=off  ADCChannel='1'  interface=None  automatic_assignment=on  address_offset=hex2dec('00')  intf_name=''  intf_description=''  default_value=0  timing_constraint=None  locs_specified=off  LOCs={}  io_standard={}  inherit_from_input=off  hdl_port=on  XmcBlockStatus=1  maskContainerNames=group4  block_type=gatewayin  block_config=sysgen:gateway_in_config  block_width_w=590  block_height_w=620  block_width=640  block_height=850
  Gate_In2 : hdlBasic/Gateway In  gui_display_data_type=Fixed-point  arith_type=Signed (2's comp)  n_bits=12  bin_pt=10  preci_type=Double  exp_width=8  frac_width=24  rows=1  columns=1  quantization="Round  (unbiased: +/- Inf)"  overflow=Saturate  period=1  UseAsADC=off  ADCChannel='1'  interface=None  automatic_assignment=on  address_offset=hex2dec('00')  intf_name=''  intf_description=''  default_value=0  timing_constraint=None  locs_specified=off  LOCs={}  io_standard={}  inherit_from_input=off  hdl_port=on  XmcBlockStatus=1  maskContainerNames=group4  block_type=gatewayin  block_config=sysgen:gateway_in_config  block_width_w=590  block_height_w=620  block_width=640  block_height=850
  Gate_out1 : hdlBasic/Gateway Out  inherit_from_input=off  hdl_port=on  rows=1  columns=1  UseAsDAC=off  DACChannel='1'  interface=None  automatic_assignment=on  address_offset=hex2dec('00')  intf_name=''  intf_description=''  timing_constraint=None  locs_specified=off  LOCs={}  io_standard={}  XmcBlockStatus=1  maskContainerNames=group4  block_type=gatewayout  block_config=sysgen:gateway_out_config  block_width_w=590  block_height_w=620  block_width=620  block_height=750
  Mux : hdlBasic/Mux  inputs=2  en=off  latency=0  precision=Full  arith_type=Unsigned  n_bits=16  bin_pt=14  quantization=Truncate  overflow=Wrap  XmcBlockStatus=1  maskContainerNames=tabcontainer1  block_type=mux  block_config=sysgen:Mux_config
  Mux1 : hdlBasic/Mux  inputs=2  en=off  latency=0  precision=Full  arith_type=Unsigned  n_bits=16  bin_pt=14  quantization=Truncate  overflow=Wrap  XmcBlockStatus=1  maskContainerNames=tabcontainer1  block_type=mux  block_config=sysgen:Mux_config
  Scale1 : hdlBasic/Scale  scale_factor=-11  XmcBlockStatus=1  maskContainerNames=group1  block_type=scale  block_config=sysgen:Scale_config
  Scale2 : hdlBasic/Scale  scale_factor=-11  XmcBlockStatus=1  maskContainerNames=group1  block_type=scale  block_config=sysgen:Scale_config
  Scale3 : hdlBasic/Scale  scale_factor=-11  XmcBlockStatus=1  maskContainerNames=group1  block_type=scale  block_config=sysgen:Scale_config
  Slice1 : hdlBasic/Slice  nbits=7  boolean_output=off  mode=Two Bit Locations  bit1=-5  base1=MSB of Input  bit0=10  base0=LSB of Input  XmcBlockStatus=1  maskContainerNames=group1  block_type=slice  block_config=sysgen:Slice_config
  Slice2 : hdlBasic/Slice  nbits=7  boolean_output=off  mode=Two Bit Locations  bit1=-5  base1=MSB of Input  bit0=10  base0=LSB of Input  XmcBlockStatus=1  maskContainerNames=group1  block_type=slice  block_config=sysgen:Slice_config
  Slice3 : hdlBasic/Slice  nbits=12  boolean_output=off  mode=Upper Bit Location + Width  bit1=-4  base1=MSB of Input  bit0=7  base0=LSB of Input  XmcBlockStatus=1  maskContainerNames=group1  block_type=slice  block_config=sysgen:Slice_config
  abs{1..6} (6 alike) : hdlBasic/Absolute  precision=Full  arith_type=Unsigned  n_bits=16  bin_pt=14  quantization=Truncate  overflow=Wrap  en=off  latency=0  XmcBlockStatus=1  maskContainerNames=tabcontainer1  block_type=abs  block_config=sysgen:Abs_config
  addsub1 : hdlBasic/AddSub  mode=Subtraction  use_carryin=off  use_carryout=off  en=off  latency=0  precision=Full  arith_type="Signed  (2's comp)"  n_bits=35  bin_pt=32  quantization="Round  (unbiased: +/- Inf)"  overflow=Saturate  use_behavioral_HDL=off  hw_selection=Fabric  pipelined=on  XmcBlockStatus=1  maskContainerNames=tabcontainer1  block_type=addsub  block_config=sysgen:Addsub_config
  addsub{2,4..6} (4 alike) : hdlBasic/AddSub  mode=Addition  use_carryin=off  use_carryout=off  en=off  latency=0  precision=Full  arith_type=Unsigned  n_bits=16  bin_pt=14  quantization="Round  (unbiased: +/- Inf)"  overflow=Saturate  use_behavioral_HDL=off  hw_selection=Fabric  pipelined=on  XmcBlockStatus=1  maskContainerNames=tabcontainer1  block_type=addsub  block_config=sysgen:Addsub_config
  addsub3 : hdlBasic/AddSub  mode=Subtraction  use_carryin=off  use_carryout=off  en=off  latency=0  precision=Full  arith_type="Signed  (2's comp)"  n_bits=35  bin_pt=32  quantization="Round  (unbiased: +/- Inf)"  overflow=Saturate  use_behavioral_HDL=off  hw_selection=Fabric  pipelined=on  XmcBlockStatus=1  maskContainerNames=tabcontainer1  block_type=addsub  block_config=sysgen:Addsub_config
  addsub7 : hdlBasic/AddSub  mode=Addition  use_carryin=off  use_carryout=off  en=off  latency=0  precision=Full  arith_type=Unsigned  n_bits=17  bin_pt=16  quantization="Round  (unbiased: +/- Inf)"  overflow=Saturate  use_behavioral_HDL=off  hw_selection=Fabric  pipelined=on  XmcBlockStatus=1  maskContainerNames=tabcontainer1  block_type=addsub  block_config=sysgen:Addsub_config
  bool1 : hdlBasic/Relational  mode=a<b  op_type=Bool  en=off  latency=0  XmcBlockStatus=1  maskContainerNames=tabcontainer1  block_type=relational  block_config=sysgen:Relational_config
  bool2 : hdlBasic/Relational  mode=a<b  op_type=Bool  en=off  latency=0  XmcBlockStatus=1  maskContainerNames=tabcontainer1  block_type=relational  block_config=sysgen:Relational_config
  Out1 : Outport
  wires:
  addsub3/1 -> abs3/1
  abs3/1 -> addsub6/1
  CMult1/1 -> addsub3/1, addsub2/1
  CMult2/1 -> addsub2/2, addsub3/2
  imx/1 -> Gate_In2/1
  rex/1 -> Gate_In1/1
  bool1/1 -> Mux/1
  addsub4/1 -> abs4/1
  abs4/1 -> addsub6/2
  Gate_In1/1 -> CMult1/1, CMult5/1, CMult3/1
  Gate_In2/1 -> CMult4/1, CMult6/1, CMult2/1
  CMult3/1 -> addsub4/1, addsub1/1
  CMult4/1 -> addsub4/2, addsub1/2
  addsub2/1 -> abs2/1
  abs2/1 -> addsub5/2
  addsub1/1 -> abs1/1
  abs1/1 -> addsub5/1
  Gate_out1/1 -> Out1/1
  Scale1/1 -> bool2/1, Mux1/2
  Mux/1 -> Mux1/3, bool2/2
  bool2/1 -> Mux1/1
  abs5/1 -> addsub7/1
  abs6/1 -> addsub7/2
  Mux1/1 -> Gate_out1/1
  Slice2/1 -> Scale2/1
  Slice1/1 -> Scale1/1
  Slice3/1 -> Scale3/1
  Scale2/1 -> bool1/1, Mux/2
  Scale3/1 -> Mux/3, bool1/2
  CMult5/1 -> abs5/1
  CMult6/1 -> abs6/1
  addsub5/1 -> Slice1/1
  addsub6/1 -> Slice2/1
  addsub7/1 -> Slice3/1
